simulink model "simulink_model1_1"  (R2014a)
settings: Solver=FixedStepDiscrete  StartTime=0.0  StopTime=10  FixedStep=0.01  RelTol=1e-3
settings Model: Creator=cya  LastModifiedBy=cya

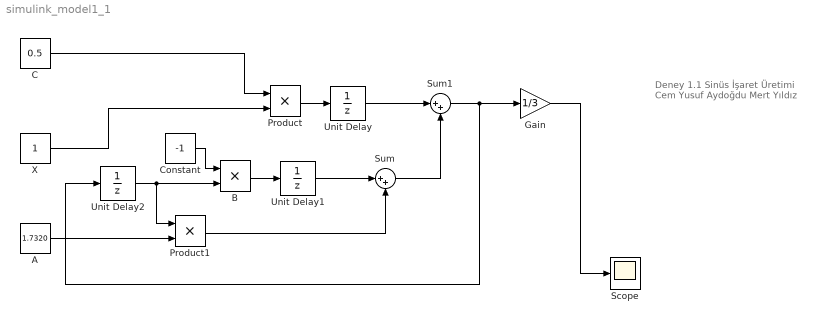
== system simulink_model1_1 ==
  note: Deney 1.1 Sinüs İşaret Üretimi
      | Cem Yusuf Aydoğdu
      | Mert Yıldız
  A : Constant  Value=1.7320
  B : Product
  C : Constant  Value=0.5
  Constant : Constant  Value=-1
  Gain : Gain  Gain=1/3
  Product : Product
  Product1 : Product
  Scope : Scope
  Sum : Sum  Inputs=|++
  Sum1 : Sum  Inputs=|++
  Unit Delay : UnitDelay  SampleTime=-1
  Unit Delay1 : UnitDelay  SampleTime=-1
  Unit Delay2 : UnitDelay  SampleTime=-1
  X : Constant
  wires:
  Sum/1 -> Sum1/2
  Constant/1 -> B/1
  B/1 -> Unit Delay1/1
  Unit Delay1/1 -> Sum/1
  Unit Delay2/1 -> Product1/1, B/2
  Product1/1 -> Sum/2
  A/1 -> Product1/2
  C/1 -> Product/1
  Product/1 -> Unit Delay/1
  X/1 -> Product/2
  Unit Delay/1 -> Sum1/1
  Sum1/1 -> Gain/1, Unit Delay2/1
  Gain/1 -> Scope/1
